simulink library "BrakeSystemLibrary"  (R2020a)
settings: Solver=VariableStepAuto  StartTime=0.0  StopTime=10.0  RelTol=1e-3
undefined symbols (not defined in the file or in its folder): BMV_Model_Relative_Error
settings Model: Creator=Jared  LastModifiedBy=Jared

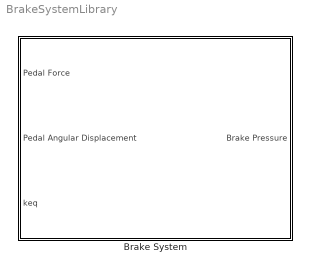
== system BrakeSystemLibrary ==
  Brake System : Subsystem

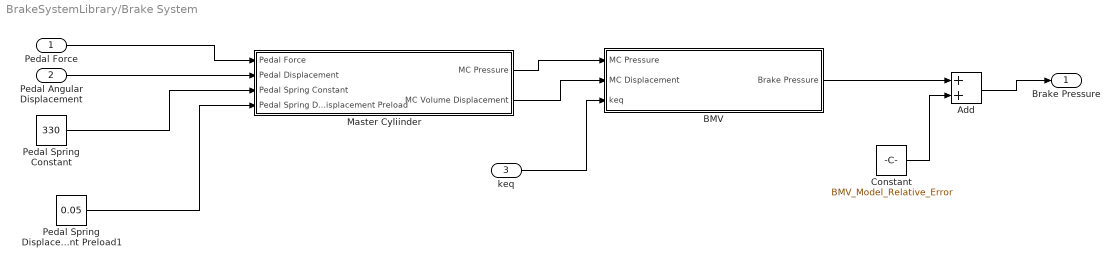
== system BrakeSystemLibrary/Brake System ==
  Pedal Force : Inport
  Pedal Angular Displacement : Inport  Port=2
  keq : Inport  Port=3
  Add : Sum
  BMV : Subsystem
  Constant : Constant  Value=BMV_Model_Relative_Error
  Master Cyliinder : Subsystem
  Pedal Spring Constant : Constant  Value=330
  Pedal Spring Displacement Preload1 : Constant  Value=0.05
  Brake Pressure : Outport
  wires:
  Master Cyliinder/1(MC Pressure) -> BMV/1(MC Pressure)
  Pedal Angular Displacement/1 -> Master Cyliinder/2(Pedal Displacement)
  Pedal Force/1 -> Master Cyliinder/1(Pedal Force)
  Master Cyliinder/2(MC Volume Displacement) -> BMV/2(MC Displacement)
  keq/1 -> BMV/3(keq)
  Pedal Spring Constant/1 -> Master Cyliinder/3(Pedal Spring Constant)
  Pedal Spring Displacement Preload1/1 -> Master Cyliinder/4(Pedal Spring Displacement Preload)
  BMV/1(Brake Pressure) -> Add/1
  Add/1 -> Brake Pressure/1
  Constant/1 -> Add/2

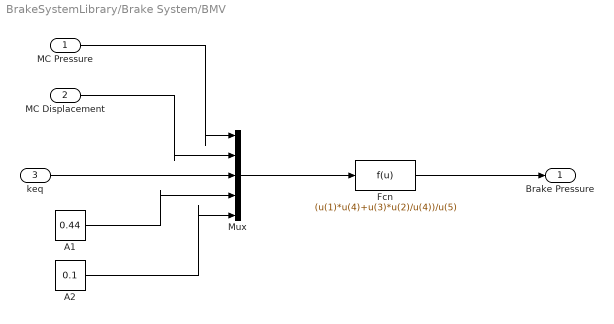
== system BrakeSystemLibrary/Brake System/BMV ==
  MC Pressure : Inport
  MC Displacement : Inport  Port=2
  keq : Inport  Port=3
  A1 : Constant  Value=0.44
  A2 : Constant  Value=0.1
  Fcn : Fcn  Expr=(u(1)*u(4)+u(3)*u(2)/u(4))/u(5)
  Mux : Mux  Inputs=5
  Brake Pressure : Outport
  wires:
  MC Displacement/1 -> Mux/2
  keq/1 -> Mux/3
  MC Pressure/1 -> Mux/1
  A2/1 -> Mux/5
  A1/1 -> Mux/4
  Mux/1 -> Fcn/1
  Fcn/1 -> Brake Pressure/1

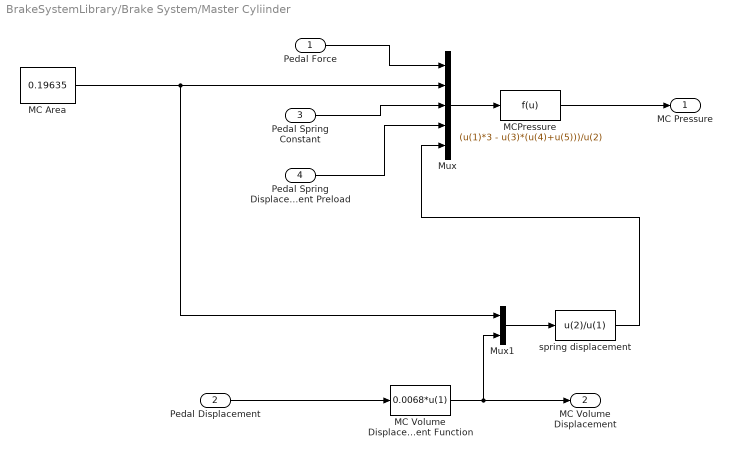
== system BrakeSystemLibrary/Brake System/Master Cyliinder ==
  Pedal Force : Inport
  Pedal Displacement : Inport  Port=2
  Pedal Spring Constant : Inport  Port=3
  Pedal Spring Displacement Preload : Inport  Port=4
  MC Area : Constant  Value=0.19635
  MC Volume Displacement Function : Fcn  Expr=0.0068*u(1)
  MCPressure : Fcn  Expr=(u(1)*3 - u(3)*(u(4)+u(5)))/u(2)
  Mux : Mux  Inputs=5
  Mux1 : Mux  Inputs=2
  spring displacement : Fcn  Expr=u(2)/u(1)
  MC Pressure : Outport
  MC Volume Displacement : Outport  Port=2
  wires:
  Pedal Displacement/1 -> MC Volume Displacement Function/1
  MCPressure/1 -> MC Pressure/1
  MC Volume Displacement Function/1 -> Mux1/2, MC Volume Displacement/1
  MC Area/1 -> Mux/2, Mux1/1
  Pedal Force/1 -> Mux/1
  Mux/1 -> MCPressure/1
  Pedal Spring Constant/1 -> Mux/3
  Mux1/1 -> spring displacement/1
  spring displacement/1 -> Mux/5
  Pedal Spring Displacement Preload/1 -> Mux/4
